simulink model "test_env"  (R2022a)
settings: Solver=VariableStepAuto  StartTime=0.0  StopTime=10  RelTol=1e-3
values from neighbouring files (symbols this model uses):
  A = [A1 A2 ... (first row only)    [main.m]
  af = 0.8    [main.m]
  ar = 1.45    [main.m]
  B = [B1 ... (first row only)    [main.m]
  dt = L_/V    (= 0.405)    [main.m]
  K = [K1 ... (first row only)    [main.m]
  L_ = ar+af    (= 2.25)    [main.m]
  V = 20/3.6    (= 5.55555555556)    [main.m]
libraries: cstblocks x1
settings Model: Creator=s393429  LastModifiedBy=s393429

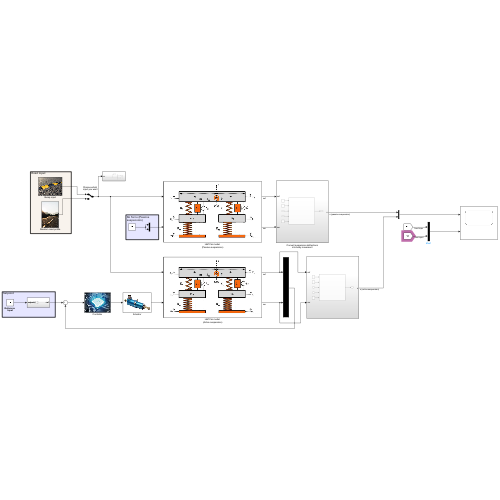
[thumbnail: Simulink's stored preview of the top-level diagram]
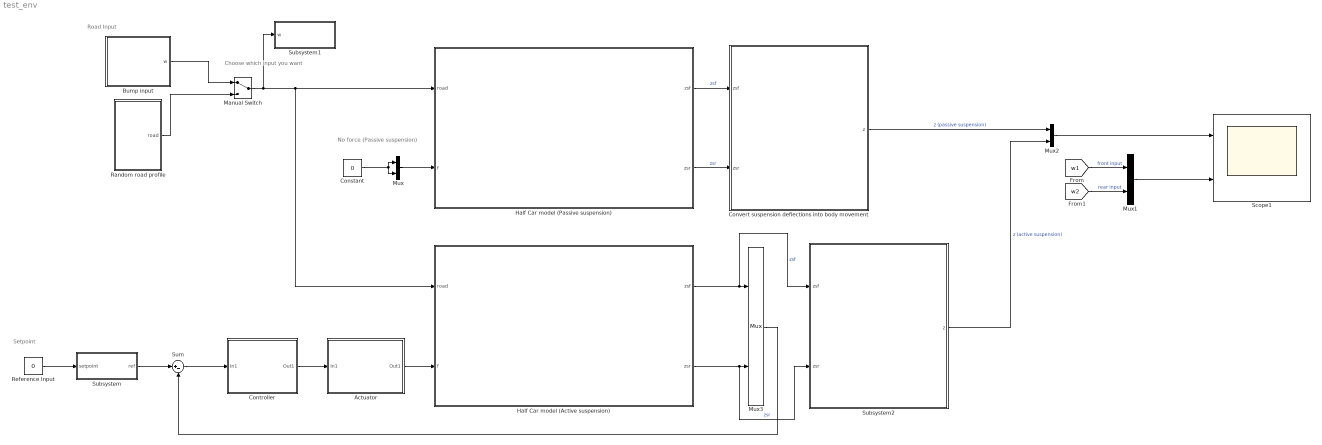
== system test_env ==
  note: Choose which
      | input you want
  note: Setpoint
  note: Road Input
  note: No force (Passive
      | suspension)
  Actuator : Subsystem
      mask Display: image('actuator.jpg'); % Use "Edit Image" on toolstrip to change.
  Bump input : Subsystem
      mask Display: image('speedbump.jpg'); % Use "Edit Image" on toolstrip to change.
  Constant : Constant  Value=0
  Controller : Subsystem
      mask Display: image('cu.jpg'); % Use "Edit Image" on toolstrip to change.
  Convert suspension deflections into body movement : Subsystem
  Half Car model (Active suspension) : Subsystem
      mask Display: image('C:\Users\s393429\OneDrive - Cranfield University\Documents\MATLAB\VCA\Assignment\icon.PNG'); % Use "Edit Image" on toolstrip to change.
  Half Car model (Passive suspension) : Subsystem
      mask Display: image('C:\Users\s393429\OneDrive - Cranfield University\Documents\MATLAB\VCA\Assignment\icon.PNG'); % Use "Edit Image" on toolstrip to change.
  Manual Switch : ManualSwitch
  Mux{,1..3} (4 alike) : Mux  Inputs=2
  Random road profile : Subsystem
      mask Display: image('road.jpg'); % Use "Edit Image" on toolstrip to change.
  Reference Input : Constant  Value=0
  Scope1 : Scope  NumInputPorts=2
  Subsystem : Subsystem
  Subsystem1 : Subsystem
  Subsystem2 : Subsystem
  Sum : Sum  Inputs=|+-
  wires:
  Constant/1 -> Mux/1, Mux/2
  Mux/1 -> Half Car model (Passive suspension)/2(f)
  Half Car model (Active suspension)/2(zsr) -> Subsystem2/2(zsr), Mux3/2  "zsr"
  Half Car model (Active suspension)/1(zsf) -> Subsystem2/1(zsf), Mux3/1  "zsf"
  Controller/1(Out1) -> Actuator/1(In1)
  Actuator/1(Out1) -> Half Car model (Active suspension)/2(f)
  Reference Input/1 -> Subsystem/1(setpoint)
  Subsystem/1(ref) -> Sum/1
  Mux3/1 -> Sum/2
  Sum/1 -> Controller/1(In1)
  Half Car model (Passive suspension)/1(zsf) -> Convert suspension deflections into body movement/1(zsf)  "zsf"
  Half Car model (Passive suspension)/2(zsr) -> Convert suspension deflections into body movement/2(zsr)  "zsr"
  Subsystem2/1(z) -> Mux2/2  "z (active suspension)"
  [w1] -> Mux1/1  "front input"
  [w2] -> Mux1/2  "rear input"
  Mux1/1 -> Scope1/2
  Mux2/1 -> Scope1/1
  Convert suspension deflections into body movement/1(z) -> Mux2/1  "z (passive suspension)"
  Bump input/1(w) -> Manual Switch/1
  Random road profile/1(road) -> Manual Switch/2
  Manual Switch/1 -> Half Car model (Passive suspension)/1(road), Half Car model (Active suspension)/1(road), Subsystem1/1(w)

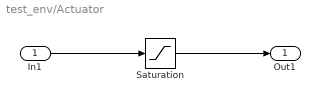
== system test_env/Actuator ==
  In1 : Inport
  Saturation : Saturate  UpperLimit=inf  LowerLimit=-inf
  Out1 : Outport
  wires:
  In1/1 -> Saturation/1
  Saturation/1 -> Out1/1

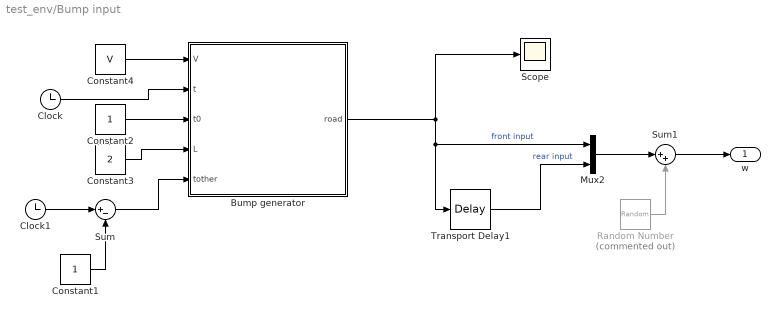
== system test_env/Bump input ==
  Bump generator : MATLAB Function  TreatAsAtomicUnit=on
  Clock : Clock
  Clock1 : Clock
  Constant1 : Constant
  Constant2 : Constant
  Constant3 : Constant  Value=2
  Constant4 : Constant  Value=V
  Mux2 : Mux  Inputs=2
  Random Number : RandomNumber  Commented=on  Variance=0.0001  SampleTime=0.1
  Scope : Scope
  Sum : Sum  Inputs=|+-
  Sum1 : Sum  Inputs=|++
  Transport Delay1 : TransportDelay  DelayTime=dt
  w : Outport
  wires:
  Constant4/1 -> Bump generator/1(V)
  Clock/1 -> Bump generator/2(t)
  Constant2/1 -> Bump generator/3(t0)
  Constant3/1 -> Bump generator/4(L)
  Bump generator/1(road) -> Mux2/1, Transport Delay1/1, Scope/1  "front input"
  Clock1/1 -> Sum/1
  Constant1/1 -> Sum/2
  Sum/1 -> Bump generator/5(tother)
  Transport Delay1/1 -> Mux2/2  "rear input"
  Mux2/1 -> Sum1/1
  Sum1/1 -> w/1
  Random Number/1 -> Sum1/2

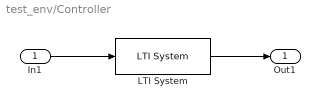
== system test_env/Controller ==
  In1 : Inport
  LTI System : cstblocks/LTI System  sys=C  IC=[]
  Out1 : Outport
  wires:
  In1/1 -> LTI System/1
  LTI System/1 -> Out1/1

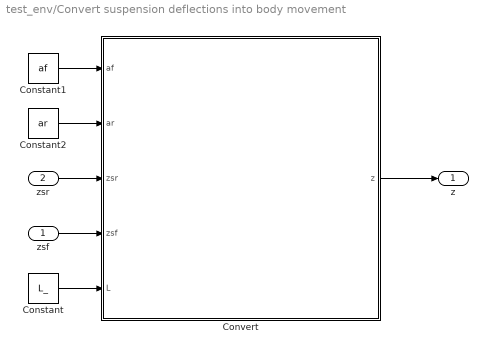
== system test_env/Convert suspension deflections into body movement ==
  zsf : Inport
  zsr : Inport  Port=2
  Constant : Constant  Value=L_
  Constant1 : Constant  Value=af
  Constant2 : Constant  Value=ar
  Convert : MATLAB Function  TreatAsAtomicUnit=on
  z : Outport
  wires:
  zsr/1 -> Convert/3(zsr)
  zsf/1 -> Convert/4(zsf)
  Constant/1 -> Convert/5(L)
  Constant1/1 -> Convert/1(af)
  Constant2/1 -> Convert/2(ar)
  Convert/1(z) -> z/1

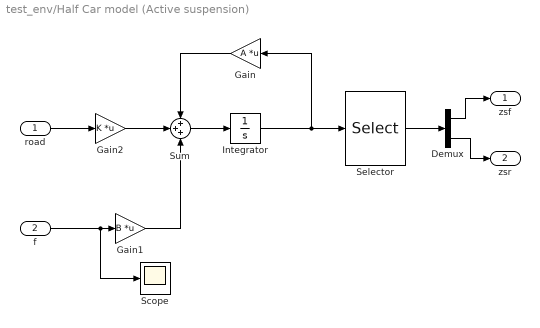
== system test_env/Half Car model (Active suspension) ==
  road : Inport
  f : Inport  Port=2
  Demux : Demux  Outputs=2
  Gain : Gain  Gain=A  Multiplication=Matrix(K*u)
  Gain1 : Gain  Gain=B  Multiplication=Matrix(K*u)
  Gain2 : Gain  Gain=K  Multiplication=Matrix(K*u)
  Integrator : Integrator
  Scope : Scope
  Selector : Selector  InputPortWidth=8  IndexOptions=Index vector (dialog)  Indices=[5 7]  OutputSizes=1
  Sum : Sum  Inputs=+++
  zsf : Outport
  zsr : Outport  Port=2
  wires:
  Integrator/1 -> Selector/1, Gain/1
  Sum/1 -> Integrator/1
  Gain/1 -> Sum/1
  f/1 -> Scope/1, Gain1/1
  Gain1/1 -> Sum/3
  road/1 -> Gain2/1
  Gain2/1 -> Sum/2
  Selector/1 -> Demux/1
  Demux/1 -> zsf/1
  Demux/2 -> zsr/1

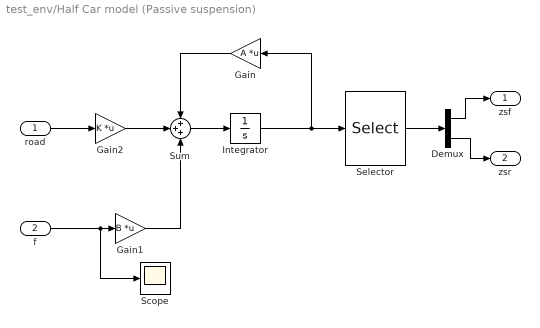
== system test_env/Half Car model (Passive suspension) ==
  road : Inport
  f : Inport  Port=2
  Demux : Demux  Outputs=2
  Gain : Gain  Gain=A  Multiplication=Matrix(K*u)
  Gain1 : Gain  Gain=B  Multiplication=Matrix(K*u)
  Gain2 : Gain  Gain=K  Multiplication=Matrix(K*u)
  Integrator : Integrator
  Scope : Scope
  Selector : Selector  InputPortWidth=8  IndexOptions=Index vector (dialog)  Indices=[5 7]  OutputSizes=1
  Sum : Sum  Inputs=+++
  zsf : Outport
  zsr : Outport  Port=2
  wires:
  Integrator/1 -> Selector/1, Gain/1
  Sum/1 -> Integrator/1
  Gain/1 -> Sum/1
  f/1 -> Scope/1, Gain1/1
  Gain1/1 -> Sum/3
  road/1 -> Gain2/1
  Gain2/1 -> Sum/2
  Selector/1 -> Demux/1
  Demux/1 -> zsf/1
  Demux/2 -> zsr/1

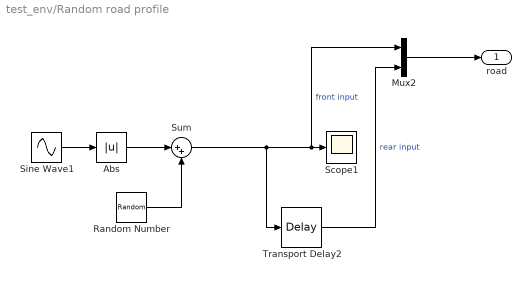
== system test_env/Random road profile ==
  Abs : Abs  SaturateOnIntegerOverflow=off
  Mux2 : Mux  Inputs=2
  Random Number : RandomNumber  Variance=.0001  SampleTime=0.01
  Scope1 : Scope
  Sine Wave1 : Sin  Amplitude=.05  Frequency=5  SampleTime=0
  Sum : Sum  Inputs=|++
  Transport Delay2 : TransportDelay  DelayTime=dt
  road : Outport
  wires:
  Mux2/1 -> road/1
  Sine Wave1/1 -> Abs/1
  Abs/1 -> Sum/1
  Transport Delay2/1 -> Mux2/2  "rear input"
  Sum/1 -> Transport Delay2/1, Mux2/1, Scope1/1  "front input"
  Random Number/1 -> Sum/2

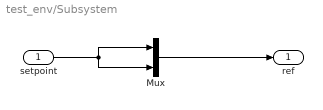
== system test_env/Subsystem ==
  setpoint : Inport
  Mux : Mux  Inputs=2
  ref : Outport
  wires:
  setpoint/1 -> Mux/1, Mux/2
  Mux/1 -> ref/1

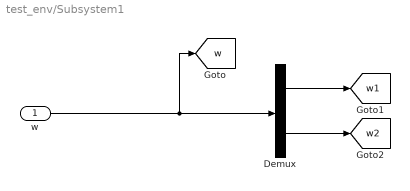
== system test_env/Subsystem1 ==
  w : Inport
  Demux : Demux  Outputs=2
  tag scope: w1=global, w2=global, w=global
  wires:
  w/1 -> [w], Demux/1
  Demux/1 -> [w1]
  Demux/2 -> [w2]

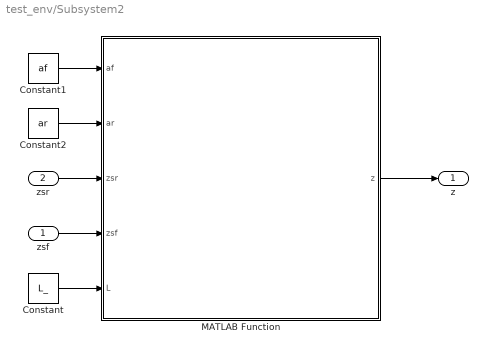
== system test_env/Subsystem2 ==
  zsf : Inport
  zsr : Inport  Port=2
  Constant : Constant  Value=L_
  Constant1 : Constant  Value=af
  Constant2 : Constant  Value=ar
  MATLAB Function : MATLAB Function  TreatAsAtomicUnit=on
  z : Outport
  wires:
  MATLAB Function/1(z) -> z/1
  Constant2/1 -> MATLAB Function/2(ar)
  Constant1/1 -> MATLAB Function/1(af)
  Constant/1 -> MATLAB Function/5(L)
  zsf/1 -> MATLAB Function/4(zsf)
  zsr/1 -> MATLAB Function/3(zsr)

== matlab function test_env/Convert suspension deflections into body movement/Convert ==
  data: af input; z output; ar input; zsr input; zsf input; L input
function z = zsrzsf2z(af, ar, zsr, zsf, L)

z = (af*zsr+ar*zsf)/L;

end

== matlab function test_env/Bump input/Bump generator ==
  data: V input; road output; t input; t0 input; L input; tother input
function road = fcn(V, t, t0, L, tother)


if t>t0 && t<=t0+L/V
        road = -1/2*0.30*(cos(2*pi*V*tother/L)-1);
else 
    road = 0;
end

end

== matlab function test_env/Subsystem2/MATLAB Function ==
  data: af input; z output; ar input; zsr input; zsf input; L input
function z = zsrzsf2z(af, ar, zsr, zsf, L)

z = (af*zsr+ar*zsf)/L;

end
